simulink model "AppDesign1"  (R2019a)
settings: Solver=VariableStepAuto  StartTime=0.0  StopTime=10.0  RelTol=1e-3
settings Model: Creator=G5  LastModifiedBy=G5

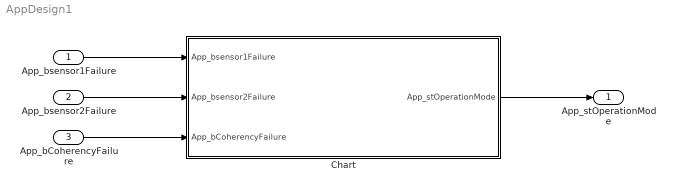
== system AppDesign1 ==
  App_bsensor1Failure : Inport
  App_bsensor2Failure : Inport  Port=2
  App_bCoherencyFailure : Inport  Port=3
  Chart : Stateflow chart  BlockKeywords=__PRM__SERIALIZED__DATA__:Stateflow Chart,Stateflow Diagram  TreatAsAtomicUnit=on
  App_stOperationMode : Outport  OutDataTypeStr=Enum: App_Modes
  wires:
  App_bsensor1Failure/1 -> Chart/1(App_bsensor1Failure)
  App_bsensor2Failure/1 -> Chart/2(App_bsensor2Failure)
  App_bCoherencyFailure/1 -> Chart/3(App_bCoherencyFailure)
  Chart/1(App_stOperationMode) -> App_stOperationMode/1

== stateflow chart AppDesign1/Chart ==
  state Normal
    en:
    App_stOperationMode = App_Modes.Normal;
  state Downgraded_1
    en:
    App_stOperationMode = App_Modes.Downgraded_Sen_1;
  state Downgraded_2
    en:
    App_stOperationMode = App_Modes.Downgraded_Sen_2;
  state Failure
    en:
    App_stOperationMode = App_Modes.Failure;
  (default) -> Normal
  (junction 10) -> Normal [order 2] : [~App_bCoherencyFailure]
  Normal -> (junction 10) : [App_bCoherencyFailure ]
  (junction 10) -> Downgraded_1 [order 1] : [App_bsensor2Failure && ~App_bsensor1Failure]
  (junction 10) -> Downgraded_2 [order 3] : [App_bsensor1Failure && ~App_bsensor2Failure]
  Downgraded_2 -> (junction 10)
  Downgraded_1 -> (junction 10)
  (junction 10) -> Failure [order 4] : [App_bCoherencyFailure]
  data: App_bsensor1Failure input; App_bsensor2Failure input; App_bCoherencyFailure input; App_stOperationMode output
